simulink model "filterbank_functest"  (R2019a)
settings: Solver=VariableStepAuto  StartTime=0.0  StopTime=4096  RelTol=1e-3
values from neighbouring files (symbols this model uses):
  d0 = input_sig(1:wideband_factor:nof_points)    [filterbank_functest_input.m]    (also in pfb_functest_deinterleave_input.m = noise_sig(1:2:end); pfb_functest_script.m = sig_2(1:wideband_factor*nof_streams:nof_points); prefilter_functest_script.m; wideband_fft_functest_script.m = real_sig(1:wideband_factor:end))
  d1 = input_sig(2:wideband_factor:nof_points)    [filterbank_functest_input.m]    (also in pfb_functest_deinterleave_input.m = real_sig(1:2:end); pfb_functest_script.m = sig_1(1:wideband_factor*nof_streams:nof_points); prefilter_functest_script.m; wideband_fft_functest_script.m = noise_sig(1:wideband_factor:end))
undefined symbols (not defined in the file or in its folder): Filterbank, PFB_FIR
libraries: xbsIndex_r4 x24
settings Model: Creator=talonm  LastModifiedBy=Ross

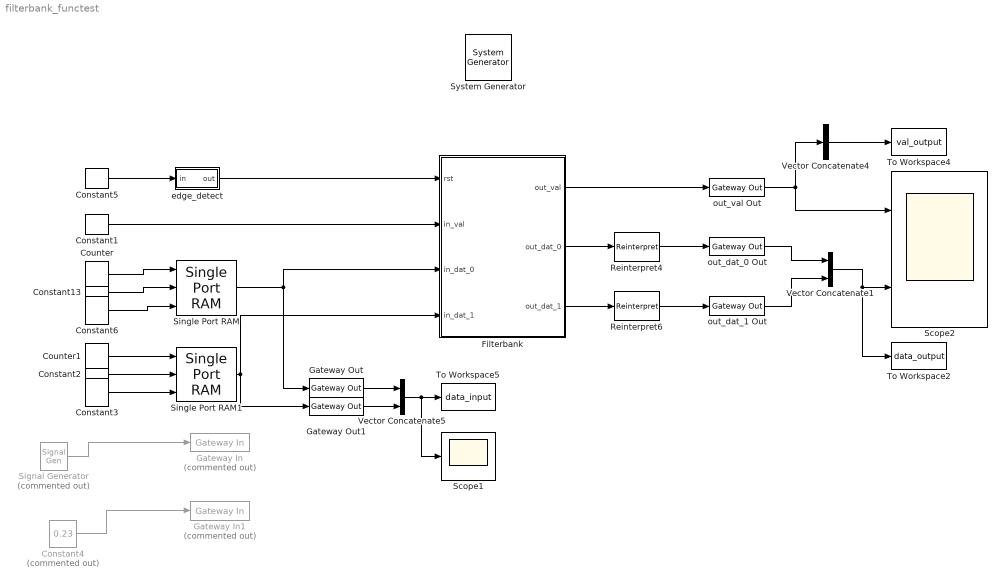
== system filterbank_functest ==
  " System Generator" : xbsIndex_r4/ System Generator  Tag=genX  xilinxfamily=kintex7  part=xc7k160t  speed=-1  package=fbg484  synthesis_tool=Vivado  clock_wrapper=Clock Enables  directory=./netlist  proj_type=Vivado  Synth_file=Vivado Synthesis Defaults  Impl_file=Vivado Implementation Defaults  testbench=on  simulink_period=1  sysclk_period=50  dcm_input_clock_period=10  incr_netlist=off  trim_vbits=Everywhere in SubSystem  dbl_ovrd=According to Block Masks  core_generation=According to Block Masks  run_coregen=off  deprecated_control=off  eval_field=0  block_type=sysgen
  Constant1 : xbsIndex_r4/Constant  const=1  gui_display_data_type=Fixed-point  arith_type=Unsigned  n_bits=1  bin_pt=0  preci_type=Single  exp_width=8  frac_width=24  explicit_period=on  period=1  equ=P=C  opselect=C  inp2=PCIN>>17  opr=+  inp1=P  carry=CIN  dbl_ovrd=off  block_type=constant
  Constant13 : xbsIndex_r4/Constant  const=0  gui_display_data_type=Fixed-point  arith_type=Signed (2's comp)  n_bits=18  bin_pt=17  preci_type=Single  exp_width=8  frac_width=24  explicit_period=off  period=1  equ=P=C  opselect=C  inp2=PCIN>>17  opr=+  inp1=P  carry=CIN  dbl_ovrd=off  block_type=constant
  Constant2 : xbsIndex_r4/Constant  const=0  gui_display_data_type=Fixed-point  arith_type=Signed (2's comp)  n_bits=18  bin_pt=17  preci_type=Single  exp_width=8  frac_width=24  explicit_period=off  period=1  equ=P=C  opselect=C  inp2=PCIN>>17  opr=+  inp1=P  carry=CIN  dbl_ovrd=off  block_type=constant
  Constant3 : xbsIndex_r4/Constant  const=0  gui_display_data_type=Boolean  arith_type=Boolean  n_bits=16  bin_pt=14  preci_type=Single  exp_width=8  frac_width=24  explicit_period=off  period=1  equ=P=C  opselect=C  inp2=PCIN>>17  opr=+  inp1=P  carry=CIN  dbl_ovrd=off  block_type=constant
  Constant4 : Constant  Commented=on  Value=0.23
  Constant5 : xbsIndex_r4/Constant  const=1  gui_display_data_type=Boolean  arith_type=Boolean  n_bits=16  bin_pt=14  preci_type=Single  exp_width=8  frac_width=24  explicit_period=on  period=1  equ=P=C  opselect=C  inp2=PCIN>>17  opr=+  inp1=P  carry=CIN  dbl_ovrd=off  block_type=constant
  Constant6 : xbsIndex_r4/Constant  const=0  gui_display_data_type=Boolean  arith_type=Boolean  n_bits=16  bin_pt=14  preci_type=Single  exp_width=8  frac_width=24  explicit_period=off  period=1  equ=P=C  opselect=C  inp2=PCIN>>17  opr=+  inp1=P  carry=CIN  dbl_ovrd=off  block_type=constant
  Counter : xbsIndex_r4/Counter  cnt_type=Free Running  cnt_to=Inf  operation=Up  start_count=0  cnt_by_val=1  arith_type=Unsigned  n_bits=6  bin_pt=0  load_pin=off  rst=off  en=off  explicit_period=on  period=1  use_behavioral_HDL=off  implementation=Fabric  dbl_ovrd=off  block_type=counter
  Counter1 : xbsIndex_r4/Counter  cnt_type=Free Running  cnt_to=Inf  operation=Up  start_count=0  cnt_by_val=1  arith_type=Unsigned  n_bits=6  bin_pt=0  load_pin=off  rst=off  en=off  explicit_period=on  period=1  use_behavioral_HDL=off  implementation=Fabric  dbl_ovrd=off  block_type=counter
  Filterbank : Subsystem  AncestorBlock=PFB_FIR/Filterbank  mask{big_endian_wb_in=off, big_endian_wb_out=off, wb_factor=2, nof_chan=1, nof_bands=128, nof_taps=4, nof_streams=1, in_dat_w=18, out_dat_w=18, coef_dat_w=18, win="hanning", fwidth=0.8, backoff_w=0, technology=Xilinx, ram_primitive="block"}
      mask prompts: big_endian_wb_in "Big endian in"; big_endian_wb_out "Big endian out"; wb_factor "Wideband factor"; nof_chan "Number of Channels"; nof_bands "Number of bands"; nof_taps "Number of taps"; nof_streams "Number of streams"; in_dat_w "Input data width"; out_dat_w "Output data width"; coef_dat_w "Coefficient data width"; win "Window function"; backoff_w "Backoff width"; technology "Vendor"; ram_primitive "Ram primitive"
      mask init:
      | Simulink.Block.eval([gcb, '/filterbank_top']);
      | 
      | fil_subsys2bb_knit();
      mask TypeOptions win: "hanning" | "hamming" | "blackman" | "bartlett"
      mask TypeOptions technology: Xilinx | UniBoard
      mask TypeOptions ram_primitive: "auto" | "block" | "ultra" | "distributed"
  Gateway In : xbsIndex_r4/Gateway In  Commented=on  gui_display_data_type=Fixed-point  arith_type="Signed  (2's comp)"  n_bits=8  bin_pt=7  preci_type=Single  exp_width=8  frac_width=24  rows=1  columns=1  quantization="Round  (unbiased: +/- Inf)"  overflow=Saturate  period=1  UseAsADC=off  ADCChannel='1'  interface=None  automatic_assignment=on  address_offset=hex2dec('00')  intf_name=''  intf_description=''  default_value=0  timing_constraint=None  locs_specified=off  LOCs={}  io_standard={}  inherit_from_input=off  hdl_port=on  dbl_ovrd=off  block_type=gatewayin
  Gateway In1 : xbsIndex_r4/Gateway In  Commented=on  gui_display_data_type=Fixed-point  arith_type="Signed  (2's comp)"  n_bits=8  bin_pt=7  preci_type=Single  exp_width=8  frac_width=24  rows=1  columns=1  quantization="Round  (unbiased: +/- Inf)"  overflow=Saturate  period=1  UseAsADC=off  ADCChannel='1'  interface=None  automatic_assignment=on  address_offset=hex2dec('00')  intf_name=''  intf_description=''  default_value=0  timing_constraint=None  locs_specified=off  LOCs={}  io_standard={}  inherit_from_input=off  hdl_port=on  dbl_ovrd=off  block_type=gatewayin
  Gateway Out : xbsIndex_r4/Gateway Out  inherit_from_input=on  hdl_port=off  rows=1  columns=1  UseAsDAC=off  DACChannel='1'  interface=None  automatic_assignment=on  address_offset=hex2dec('00')  intf_name=''  intf_description=''  timing_constraint=None  locs_specified=off  LOCs={}  io_standard={}  block_type=gatewayout
  Gateway Out1 : xbsIndex_r4/Gateway Out  inherit_from_input=on  hdl_port=off  rows=1  columns=1  UseAsDAC=off  DACChannel='1'  interface=None  automatic_assignment=on  address_offset=hex2dec('00')  intf_name=''  intf_description=''  timing_constraint=None  locs_specified=off  LOCs={}  io_standard={}  block_type=gatewayout
  Reinterpret4 : xbsIndex_r4/Reinterpret  force_arith_type=on  arith_type="Signed  (2's comp)"  force_bin_pt=on  bin_pt=17  block_type=reinterpret
  Reinterpret6 : xbsIndex_r4/Reinterpret  force_arith_type=on  arith_type="Signed  (2's comp)"  force_bin_pt=on  bin_pt=17  block_type=reinterpret
  Scope1 : Scope
  Scope2 : Scope  NumInputPorts=2
  Signal Generator : SignalGenerator  Commented=on  Frequency=0.5  Units=rad/sec
  Single Port RAM : xbsIndex_r4/Single Port RAM  depth=64  initVector=[d0]  distributed_mem=Block RAM  write_mode=Read After Write  rst=off  init_reg=0  en=off  optimize_latency=off  latency=1  optimize=Area  dbl_ovrd=off  simulation_type=fast_sim  block_type=spram
  Single Port RAM1 : xbsIndex_r4/Single Port RAM  depth=64  initVector=[d1]  distributed_mem=Block RAM  write_mode=Read After Write  rst=off  init_reg=0  en=off  optimize_latency=off  latency=1  optimize=Area  dbl_ovrd=off  simulation_type=fast_sim  block_type=spram
  To Workspace2 : ToWorkspace  VariableName=data_output  SaveFormat=Timeseries  SampleTime=-1
  To Workspace4 : ToWorkspace  VariableName=val_output  SaveFormat=Timeseries  SampleTime=-1
  To Workspace5 : ToWorkspace  VariableName=data_input  SaveFormat=Timeseries  SampleTime=-1
  Vector Concatenate1 : Concatenate
  Vector Concatenate4 : Concatenate  NumInputs=1
  Vector Concatenate5 : Concatenate
  edge_detect : Subsystem  AncestorBlock=casper_library_misc/edge_detect  mask(edge_detect){edge=Rising, polarity=Active High, x_in=[0 0.08 0.08 0.16 0.16 0.24 0.24 0.32 0.32 0.4], y_in=[-1 -1  1  1  1  1  1  1  1  1], x_out=[0.6 0.68 0.68 0.76 0.76 0.84 0.84 0.92 0.92 1], y_out=[-1 -1  1  1 -1 -1 -1 -1 -1 -1]}
      mask prompts: edge "Edge Type"; polarity "Output Polarity"; x_in "Input X Positions"; y_in "Input Y Positions"; x_out "Output X Positions"; y_out "Output Y Positions"
      mask help: Output is active for one-cycle after each edge of the specified type (i.e. rising, falling or both).
      mask init:
      | edge_detect_init(gcb,...
      |     'edge',edge,...
      |     'polarity',polarity,...
      |     'x_in',x_in,...
      |     'x_out',x_out,...
      |     'y_in',y_in,...
      |     'y_out',y_out);
      | 
      | x_in_num=str2num(getfield(getfield(get_param(gcb,'UserData'),'parameters'),'x_in'));
      | x_out_num=str2num(getfield(getfield(get_param(gcb,'UserData'),'parameters'),'x_out'));
      | y_in_num=str2num(getfield(getfield(get_param(gcb,'UserData'),'parameters'),'y_in'));
      | y_out_num=str2num(getfield(getfield(get_param(gcb,'UserData'),'parameters'),'y_out'));
      settings: AttributesFormatString=|
      | rising edges
      | active high
      mask Help: Output is active for one-cycle after each edge of the specified type (i.e. rising, falling, or both).  Latency is zero.
      mask TypeOptions edge: Rising | Falling | Both
      mask TypeOptions polarity: Active High | Active Low
      mask Display:
      | plot(x_in_num,0.5+y_in_num*0.2);
      | plot(x_out_num,0.5+y_out_num*0.2);
  out_dat_0 Out : xbsIndex_r4/Gateway Out  inherit_from_input=on  hdl_port=off  rows=1  columns=1  UseAsDAC=off  DACChannel='1'  interface=None  automatic_assignment=on  address_offset=hex2dec('00')  intf_name=''  intf_description=''  timing_constraint=None  locs_specified=off  LOCs={}  io_standard={}  block_type=gatewayout
  out_dat_1 Out : xbsIndex_r4/Gateway Out  inherit_from_input=on  hdl_port=off  rows=1  columns=1  UseAsDAC=off  DACChannel='1'  interface=None  automatic_assignment=on  address_offset=hex2dec('00')  intf_name=''  intf_description=''  timing_constraint=None  locs_specified=off  LOCs={}  io_standard={}  block_type=gatewayout
  out_val Out : xbsIndex_r4/Gateway Out  inherit_from_input=on  hdl_port=off  rows=1  columns=1  UseAsDAC=off  DACChannel='1'  interface=None  automatic_assignment=on  address_offset=hex2dec('00')  intf_name=''  intf_description=''  timing_constraint=None  locs_specified=off  LOCs={}  io_standard={}  block_type=gatewayout
  wires:
  Filterbank/2(out_dat_0) -> Reinterpret4/1
  Filterbank/1(out_val) -> out_val Out/1
  Reinterpret4/1 -> out_dat_0 Out/1
  out_val Out/1 -> Vector Concatenate4/1, Scope2/1
  Constant6/1 -> Single Port RAM/3
  Constant13/1 -> Single Port RAM/2
  Counter/1 -> Single Port RAM/1
  Reinterpret6/1 -> out_dat_1 Out/1
  Vector Concatenate4/1 -> To Workspace4/1
  Signal Generator/1 -> Gateway In/1
  Constant4/1 -> Gateway In1/1
  Gateway Out/1 -> Vector Concatenate5/1
  Vector Concatenate5/1 -> Scope1/1, To Workspace5/1
  Constant5/1 -> edge_detect/1(in)
  edge_detect/1(out) -> Filterbank/1(rst)
  Single Port RAM1/1 -> Gateway Out1/1, Filterbank/4(in_dat_1)
  Vector Concatenate1/1 -> To Workspace2/1, Scope2/2
  out_dat_0 Out/1 -> Vector Concatenate1/1
  out_dat_1 Out/1 -> Vector Concatenate1/2
  Constant3/1 -> Single Port RAM1/3
  Constant2/1 -> Single Port RAM1/2
  Counter1/1 -> Single Port RAM1/1
  Gateway Out1/1 -> Vector Concatenate5/2
  Constant1/1 -> Filterbank/2(in_val)
  Single Port RAM/1 -> Gateway Out/1, Filterbank/3(in_dat_0)
  Filterbank/3(out_dat_1) -> Reinterpret6/1

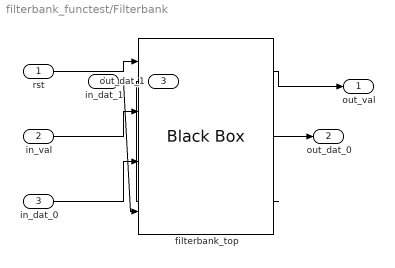
== system filterbank_functest/Filterbank ==
  rst : Inport  SampleTime=1
  in_val : Inport  Port=2
  in_dat_0 : Inport  Port=3
  in_dat_1 : Inport  Port=4
  filterbank_top : xbsIndex_r4/Black Box  init_code=filterbank_top_config  sim_method=ISE Simulator  verbose=off  block_type=blackbox2
  out_val : Outport
  out_dat_0 : Outport  Port=2
  out_dat_1 : Outport  Port=3
  wires:
  in_val/1 -> filterbank_top/2
  rst/1 -> filterbank_top/1
  in_dat_0/1 -> filterbank_top/3
  filterbank_top/1 -> out_val/1
  filterbank_top/2 -> out_dat_0/1
  in_dat_1/1 -> filterbank_top/4
  filterbank_top/3 -> out_dat_1/1

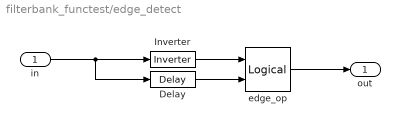
== system filterbank_functest/edge_detect ==
  in : Inport
  Delay : xbsIndex_r4/Delay  rst=off  infoeditControl=Selection of Reset will increase slice count due to use of real FFs and instead of SRLs  en=off  latency=1  reg_retiming=off  dbl_ovrd=off  block_type=delay
      settings: xl_area=[0, 0, 0, 0, 0, 0, 0]
  Inverter : xbsIndex_r4/Inverter  en=off  latency=0  dbl_ovrd=off  block_type=inv
      settings: xl_area=[0, 0, 0, 0, 0, 0, 0]
  edge_op : xbsIndex_r4/Logical  logical_function=NOR  inputs=2  en=off  latency=0  precision=Full  arith_type=Unsigned  n_bits=8  bin_pt=2  align_bp=on  dbl_ovrd=off  block_type=logical
      settings: xl_area=[0, 0, 0, 0, 0, 0, 0]
  out : Outport
  wires:
  Inverter/1 -> edge_op/1
  edge_op/1 -> out/1
  in/1 -> Inverter/1, Delay/1
  Delay/1 -> edge_op/2
